simulink library "relay_modbus_lib"  (Simulink 8.1)
settings: Solver=ode45  StartTime=0.0  StopTime=10.0  RelTol=1e-3
undefined symbols (not defined in the file or in its folder): Ts
undefined symbols (not defined in the file): F4
libraries: simulink_extras x9, simulink x5, relay_PLL_lib x3, RMS_lib x3, powerlib_extras x2, relay_ANSI_functions_lib x2, relay_PQSPF_lib x1, relay_ANSI_F25_lib x1, relay_mgc_cmd_lib x1, relay_tripOutMng_lib x1
settings Model: Creator=RE25624  LastModifiedBy=hptb1

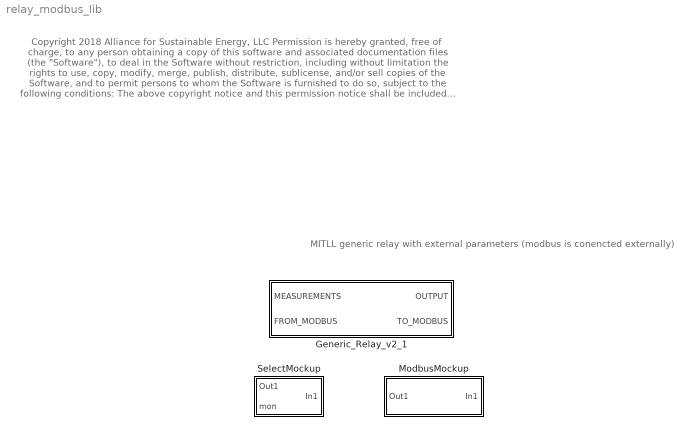
== system relay_modbus_lib ==
  note: MITLL generic relay with external parameters (modbus is conencted externally)
  note: Copyright 2018 Alliance for Sustainable Energy, LLC
      |
      | Permission is hereby granted, free of charge, to any person obtaining a copy of this software
      | and associated documentation files (the "Software"), to deal in the Software without restriction,
      | including without limitation the rights to use, copy, modify, merge, publish, distribute, sublicense,
      | and/or sell copies of the Software, and to permit persons to whom the Software is furnished to do so,
      | subject to the following conditions:
      |
      | The above copyright notice and this permission notice shall be included in all copies or substantial portions of the Software.
      |
      | THE SOFTWARE IS PROVIDED "AS IS", WITHOUT WARRANTY OF ANY KIND, EXPRESS OR IMPLIED, INCLUDING
      | BUT NOT LIMITED TO THE WARRANTIES OF MERCHANTABILITY, FITNESS FOR A PARTICULAR PURPOSE AND
      | NONINFRINGEMENT. IN NO EVENT SHALL THE AUTHORS, THE COPYRIGHT HOLDERS, THE UNITED STATES,
      | THE UNITED STATES DEPARTMENT OF ENERGY, OR ANY OF THEIR EMPLOYEES BE LIABLE FOR ANY CLAIM,
      | DAMAGES OR OTHER LIABILITY, WHETHER IN AN ACTION OF CONTRACT, TORT OR OTHERWISE, ARISING FROM,
      | OUT OF OR IN CONNECTION WITH THE SOFTWARE OR THE USE OR OTHER DEALINGS IN THE SOFTWARE.
  Generic_Relay_v2_1 : Subsystem  mask(Generic Relay){Ts=Ts, relay_settings=[F4(1,:)]}
      mask prompts: Ts "Sampling Time [Sec]"; relay_settings "Relay Settings"
      mask help:
      | This relay simulates functions: synchronizing or synchronism-check (25), phase instantaneous overcurrent (50P), AC inverse time overcurrent (51P), undervoltage relay (27), and overvoltage relay (59).
      |
      | FEATURES:
      | 1) Receives commands from the microgrid controller via MODBUS/TCP
      | 2) Two groups of interchangeable protection settings
      |     - To be used for grid-tied and islanded protection modes
      | 3) Locked-out only enabled for functions (50P), (51P)
      |     - (27) and (59) pickups will be model inputs for the next revision
      | 4) MODBUS commands expected in the following order:
      |    a) Functions reset (Holding Reg# 2000)
      |    b) Breaker state   (Holding Reg# 2001)
      |    c) Protection mode (Holding Reg# 2002)
      |       - bit = 0; parameter group#1 (default)
      |       - bit = 1; parameter group#2
      |
      | See help or integration packet for further information.
      mask Help:
      | Procedure to reclose a breaker:
      | 1) reset all functions (Holding Reg# 2000)
      | 2) set breaker state (Holding Reg# 2001) to generate a close signal
      | 	- Synch-check (25) will automatically activate
      | 	- bit = 0, trip functions are active
      | 	- bit = 1, trip functions are not active
      | 
      | 
      | 
      | Field format/order for relay settings:
      | 	- Assuming zero delay between group settings changes
      | 
      | 1.  Relay#
      | 2.  Nominal VRMSLL
      | 3.  Max. Slip Voltage [%]
      | 4.  Max. Slip Angle [degree]
      | 5.  Max. Slip Frequency [Hz]
      | 6.  27P and 59P Trip Delay [Sec]
      | 7.  CT Primary
      | 
      | Parameter Group #1
      | 8.  50P Instantaneous overcurrent (IOC) Trip Pickup
      | 9.  50P IOC Trip Delay [sec]
      | 10.  51P Time overcurrent (TOC) Trip Pickup
      | 11.  51P Curve Type
      | 12.  51P TOC Time Dial
      | 13.  27P Trip Pickup [pu]
      | 14.  59P Trip Pickup [pu]
      | 
      | Parameter Group #2
      | 15.  50P IOC Trip Pickup
      | 16.  50P IOC Trip Delay [sec]
      | 17.  51P TOC Trip Pickup
      | 18.  51P Curve Type
      | 19.  51P TOC Time Dial
      | 20.  27P Trip Pickup [pu]
      | 21.  59P Trip Pickup [pu]
      | 
      | Available TCC Characteristics:
      | 	- The degree of inverseness for each curve approximates SEL-751
      | 
      | 51P Curve
      | 1: moderate inverse
      | 2: inverse
      | 3: very inverse
      | 4: extremely inverse
      | 
      | References:
      | [1] IEEE Std. C37.112-1996
      | [2] SEL 751 Instruction manual
      | [3] MIT-LL 2nd Microgrid Controller Symposium - Integration Packet
  ModbusMockup : Subsystem
  SelectMockup : Subsystem  mask{sigID=1, sigN=6}
      mask prompts: sigID "Signal ID"; sigN "Signals count"
      mask Display: disp(['Select signal\n' num2str(sigID) '/' num2str(sigN)]);

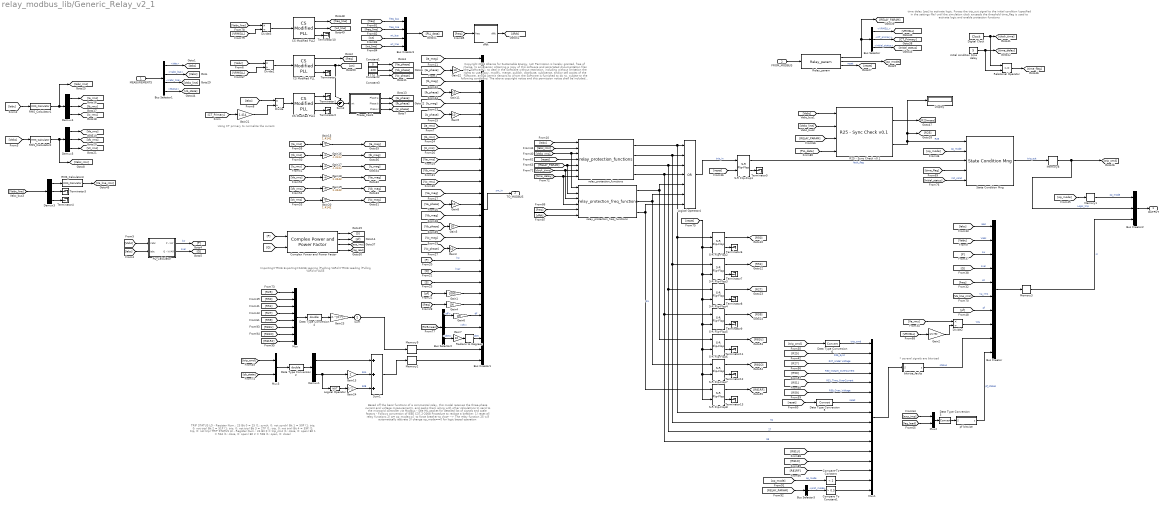
== system relay_modbus_lib/Generic_Relay_v2_1 ==
  note: Importing=TRUE
      | Exporting=FALSE
      |
      | Lagging (Pushing VARs)=TRUE
      | Leading (Pulling VARs)=FALSE
  note: * several signals are bitwised
  note: Using CT primary to normalize the current.
  note: TRIP STATUS LO - Register Num.: 23
      | Bit 0 = 25  (1: synch, 0: not synch)
      | Bit 1 = 50P (1: trip, 0: not trip)
      | Bit 2 = 51P (1: trip, 0: not trip)
      | Bit 3 = 27P (1: trip, 0: not trip)
      | Bit 4 = 59P (1: trip, 0: not trip)
      |
      | TRIP STATUS HI - Register Num.: 24
      | Bit 0 = trip_cmd  (1: close, 0: open)
      | Bit 1 = 52A (1: close, 0: open)
      | Bit 2 = 52B (1: open, 0: close)
  note: Based off the basic functions of a commercial relay, this model receives
      | the three-phase current and voltage measurements, and packs
      | them along with other calculations to send to the microgrid
      | controller via Modbus
      |
      | - See HIL packet for detailed list of signals and scale factors
      | - Follows convention of IEEE C37.2-2008
      |
      | Procedure to reclose a breaker:
      | 1) reset all relay functions
      | 2) set op_mode==1 to force breaker to close
      |    --> The relay function 25 will automatically activate
      | 3) change op_mode==0 for logic based operation
  note: time delay [sec] to activate logic. Forces the trip_out signal to the initial condition
      | (specified in the settings file) until the simulation clock exceeds the threshold
      |
      | time_flag is used to activate logic and enable protection functions
  note: Copyright 2018 Alliance for Sustainable Energy, LLC
      |
      | Permission is hereby granted, free of charge, to any person obtaining a copy of this software
      | and associated documentation files (the "Software"), to deal in the Software without restriction,
      | including without limitation the rights to use, copy, modify, merge, publish, distribute, sublicense,
      | and/or sell copies of the Software, and to permit persons to whom the Software is furnished to do so,
      | subject to the following conditions:
      |
      | The above copyright notice and this permission notice shall be included in all copies or substantial portions of the Software.
      |
      | THE SOFTWARE IS PROVIDED "AS IS", WITHOUT WARRANTY OF ANY KIND, EXPRESS OR IMPLIED, INCLUDING
      | BUT NOT LIMITED TO THE WARRANTIES OF MERCHANTABILITY, FITNESS FOR A PARTICULAR PURPOSE AND
      | NONINFRINGEMENT. IN NO EVENT SHALL THE AUTHORS, THE COPYRIGHT HOLDERS, THE UNITED STATES,
      | THE UNITED STATES DEPARTMENT OF ENERGY, OR ANY OF THEIR EMPLOYEES BE LIABLE FOR ANY CLAIM,
      | DAMAGES OR OTHER LIABILITY, WHETHER IN AN ACTION OF CONTRACT, TORT OR OTHERWISE, ARISING FROM,
      | OUT OF OR IN CONNECTION WITH THE SOFTWARE OR THE USE OR OTHER DEALINGS IN THE SOFTWARE.
  MEASUREMENTS : Inport
  FROM_MODBUS : Inport  Port=2
  Bus Creator : BusCreator  Inputs=10
  Bus Creator1 : BusCreator  Inputs=28
  Bus Creator2 : BusCreator  Inputs=3
  Bus Creator3 : BusCreator
  Bus Selector : BusSelector  OutputSignals=VRMSLL,CT_primary,Initial_status
  Bus Selector1 : BusSelector  OutputSignals=Iabc,Vabc_bus,Vabc_line,Status
  Bus Selector2 : BusSelector  OutputSignals=dF,dV,dWt
  Bus Selector3 : BusSelector  OutputSignals=prot_mode
  CS Modified PLL : relay_PLL_lib/CS Modified PLL  Flim=[55 66]  Par_Init=[0 60]  ParK=[ 180 3200 1 ]  Ts=Ts  AGC=off
  CS Modified PLL1 : relay_PLL_lib/CS Modified PLL  Flim=[55 66]  Par_Init=[0 60]  ParK=[ 180 3200 1 ]  Ts=Ts  AGC=off
  CS Modified PLL2 : relay_PLL_lib/CS Modified PLL  Flim=[55 66]  Par_Init=[0 60]  ParK=[ 180 3200 1 ]  Ts=Ts  AGC=off
  Compare To Constant : simulink/Logic and Bit Operations/Compare To Constant  relop=<  const=2  OutDataTypeStr=boolean
  Compare To Constant1 : simulink/Logic and Bit Operations/Compare To Constant  relop=>  const=0.5  OutDataTypeStr=boolean
  Complex Power and Power Factor : relay_PQSPF_lib/Complex Power and Power Factor
  Constant1 : Constant  Value=0
  Constant2 : Constant  Value=-120
  Constant3 : Constant  Value=120
  Data Type Conversion2 : DataTypeConversion  OutDataTypeStr=double
  Data Type Conversion3 : DataTypeConversion
  Data Type Conversion4 : DataTypeConversion  OutDataTypeStr=double
  Data Type Conversion5 : DataTypeConversion
  Data Type Conversion6 : DataTypeConversion
  Demux1 : Demux  Outputs=2
  Demux3 : Demux  Outputs=3
  Demux4 : Demux  Outputs=3
  Demux5 : Demux  Outputs=3
  Digital Clock : DigitalClock  SampleTime=Ts
  Display : Display
  Divide{,1..3} (4 alike) : Product  Inputs=*/
  Gain1 : Gain  Gain=1000
  Gain{3,5,7..9,11..12} (7 alike) : Gain  Gain=10
  Gain13 : Gain  Gain=2
  Gain{15..20} (6 alike) : Gain  Gain=1.4142
  Gain2 : Gain  Gain=1/1.732
  Gain21 : Gain  Gain=1.414
  Gain23 : Gain  Gain=2.^[0:7]
  Gain24 : Gain  Gain=2^2
  Gain4 : Gain  Gain=100
  Gain6 : Gain  Gain=100
  Logical Operator : Logic  Operator=NOT  AllPortsSameDT=off  OutDataTypeStr=boolean
  Logical Operator4 : Logic  Operator=OR  Inputs=7  AllPortsSameDT=off  OutDataTypeStr=boolean
  Memory{1..3,8..9} (5 alike) : Memory
  Mux : Mux  Inputs=8
  Mux1 : Mux  Inputs=16
  Mux2 : Mux  Inputs=2
  Mux3 : Mux  Inputs=2
  PQ_Calculator : Subsystem
  Phase_Calc1 : Subsystem
  R25 - Sync Check v0.1 : relay_ANSI_F25_lib/R25 - Sync Check v0.1  Ts=Ts
  RMS_Calculator1 : RMS_lib/RMS_Calculator  Ts=Ts
  RMS_Calculator2 : RMS_lib/RMS_Calculator  Ts=Ts
  RMS_Calculator3 : RMS_lib/RMS_Calculator  Ts=Ts
  Radians to Degrees : simulink_extras/Transformations/Radians to Degrees
  Relational Operator : RelationalOperator  OutDataTypeStr=boolean
  Relay_param : relay_mgc_cmd_lib/Relay_param  relay_settings=relay_settings
  S-R Flip-Flop{1..8} (8 alike) : simulink_extras/Flip Flops/S-R Flip-Flop  initial_condition=0
  State Condition Mng : relay_tripOutMng_lib/State Condition Mng
  Sum : Sum  Inputs=+
  Sum1 : Sum  Inputs=+++
  Sum2 : Sum  Inputs=-+|
  Terminator{,1..13} (14 alike) : Terminator
  bitwise_faults : Subsystem
  dfdt : Subsystem
  initial condition time delay : Constant  Value=5
  pf bitwise : Subsystem
  relay_protection_freq_functions : relay_ANSI_functions_lib/relay_protection_freq_functions  Ts=Ts
  relay_protection_functions : relay_ANSI_functions_lib/relay_protection_functions  Ts=Ts
  OUTPUT : Outport
  TO_MODBUS : Outport  Port=2
  wires:
  Gain23/1 -> Sum/1
  [R81RF] -> Mux/8
  [R81O] -> Mux/7
  [R81U] -> Mux/6
  Compare To Constant1/1 -> Mux1/16
  Bus Selector3/1 -> Compare To Constant1/1  "<prot_mode>"
  [RELAY_PARAM] -> Bus Selector3/1
  Compare To Constant/1 -> Mux1/15
  [op_mode] -> Compare To Constant/1  "op_mode"
  [R81RF] -> Mux1/14
  [R81O] -> Mux1/13
  [R81U] -> Mux1/12
  relay_protection_freq_functions/2 -> S-R Flip-Flop7/1, Logical Operator4/6
  relay_protection_freq_functions/1 -> Logical Operator4/5, S-R Flip-Flop6/1
  S-R Flip-Flop6/1 -> [R81U]
  S-R Flip-Flop7/1 -> [R81O]
  S-R Flip-Flop8/1 -> [R81RF]
  S-R Flip-Flop8/2 -> Terminator13/1
  S-R Flip-Flop7/2 -> Terminator12/1
  S-R Flip-Flop6/2 -> Terminator11/1
  [reset] -> S-R Flip-Flop2/2, S-R Flip-Flop3/2, S-R Flip-Flop4/2, S-R Flip-Flop5/2, S-R Flip-Flop6/2, S-R Flip-Flop7/2, S-R Flip-Flop8/2
  relay_protection_freq_functions/3 -> Logical Operator4/7, S-R Flip-Flop8/1  "51"
  [dfdt] -> relay_protection_freq_functions/6
  [freq] -> relay_protection_freq_functions/5
  dfdt/1(dfdt) -> [dfdt]
  [freq] -> dfdt/1(freq)
  [wt_line] -> Bus Creator3/4  "wt_line"
  [wt] -> Bus Creator3/3  "wt_bus"
  [freq_line] -> Bus Creator3/2  "freq_line"
  [freq] -> Bus Creator3/1  "freq_bus"
  Bus Creator3/1 -> [PLL_data]
  [PLL_data] -> R25 - Sync Check v0.1/4
  CS Modified PLL2/3 -> Terminator10/1
  CS Modified PLL2/2 -> [wt_line]
  CS Modified PLL2/1 -> [freq_line]
  Divide3/1 -> CS Modified PLL2/1
  [VRMSLL] -> Divide3/2
  [Vabc_line] -> Divide3/1
  Radians to Degrees/1 -> Bus Creator1/26  "dWt"
  Gain7/1 -> Radians to Degrees/1
  Gain6/1 -> Bus Creator1/24  "dF"
  Bus Selector2/3 -> Gain7/1  "<dWt>"
  Bus Selector2/1 -> Gain6/1  "<dF>"
  Bus Selector2/2 -> Bus Creator1/25  "<dV>"
  [R25meas] -> Bus Selector2/1
  R25 - Sync Check v0.1/1 -> [R25meas]
  relay_protection_functions/1 -> Logical Operator4/1, S-R Flip-Flop2/1, Mux1/8
  [S] -> Bus Creator1/21
  [Q] -> Bus Creator1/20  "kvar"
  [P] -> Bus Creator1/19  "kw"
  Sum2/1 -> Phase_Calc1/1(wt)
  S-R Flip-Flop2/1 -> [R50]
  S-R Flip-Flop3/1 -> [R51]
  S-R Flip-Flop4/1 -> [R27]
  S-R Flip-Flop5/1 -> [R59]
  S-R Flip-Flop5/2 -> Terminator9/1
  S-R Flip-Flop4/2 -> Terminator8/1
  S-R Flip-Flop3/2 -> Terminator7/1
  S-R Flip-Flop2/2 -> Terminator6/1
  RMS_Calculator3/1 -> [Va_line_rms]
  [Vabc_line] -> Demux3/1
  Relational Operator/1 -> [time_flag]
  Demux3/3 -> Terminator4/1
  Demux3/2 -> Terminator3/1
  Demux3/1 -> RMS_Calculator3/1
  Gain2/1 -> Divide2/2
  Logical Operator/1 -> Gain24/1
  [Initial_status] -> State Condition Mng/5  "init_cond"
  Bus Selector/3 -> [Initial_status]  "<Initial_status>"
  [time_delay] -> relay_protection_freq_functions/4, relay_protection_functions/7
  [clock_time] -> relay_protection_freq_functions/3, relay_protection_functions/6
  Relay_param/3 -> [reset]  "reset"
  initial condition time delay/1 -> [time_delay], Relational Operator/2
  [time_flag] -> State Condition Mng/4
  Digital Clock/1 -> [clock_time], Relational Operator/1
  Gain21/1 -> Divide/2
  Relay_param/2 -> [op_mode]
  [Va_rms] -> Divide2/1
  [VRMSLL] -> Gain2/1
  [VRMSLL] -> Divide1/2
  Divide1/1 -> CS Modified PLL/1
  [Vabc] -> Divide1/1
  Bus Selector/1 -> [VRMSLL]  "<VRMSLL>"
  [RELAY_PARAM] -> R25 - Sync Check v0.1/3
  [RELAY_PARAM] -> relay_protection_freq_functions/2, relay_protection_functions/5
  [Iabc] -> relay_protection_functions/1
  [Vabc_rms] -> relay_protection_freq_functions/1, relay_protection_functions/3
  [Iabc_rms] -> relay_protection_functions/2
  [reset] -> relay_protection_functions/4
  Relay_param/1 -> Bus Selector/1, [RELAY_PARAM]
  Bus Selector/2 -> [CT_Primary]  "<CT_primary>"
  Data Type Conversion3/1 -> pf bitwise/1(S)
  Memory3/1 -> Bus Creator2/3  "m"
  [lag_lead] -> Mux2/2
  [exp_imp] -> Mux2/1
  pf bitwise/1(s) -> Bus Creator/10  "pf_states"
  Mux2/1 -> Data Type Conversion3/1
  Complex Power and Power Factor/4 -> [lag_lead]
  Complex Power and Power Factor/3 -> [exp_imp]
  Complex Power and Power Factor/2 -> [pf]
  Complex Power and Power Factor/1 -> [S]
  [Q] -> Complex Power and Power Factor/2
  [P] -> Complex Power and Power Factor/1
  Bus Creator2/1 -> OUTPUT/1
  Memory1/1 -> Bus Creator2/1  "op_mode"
  Bus Creator/1 -> Memory3/1
  MEASUREMENTS/1 -> Bus Selector1/1
  Bus Selector1/3 -> [Vabc_line]  "<Vabc_line>"
  Bus Selector1/2 -> [Vabc]  "<Vabc_bus>"
  Bus Selector1/1 -> [Iabc]  "<Iabc>"
  [Vabc_line] -> R25 - Sync Check v0.1/2
  Data Type Conversion6/1 -> Mux1/1  "trip_cmd"
  Data Type Conversion5/1 -> Mux1/7  "reset"
  [R59] -> Mux1/6  "R59_Over_Voltage"
  [R51] -> Mux1/5  "R51_Time_OverCurrent"
  [R50] -> Mux1/4  "R50_Instant_OverCurrent"
  [R27] -> Mux1/3  "R27_Under Voltage"
  [R25] -> Mux1/2  "R25_Sync"
  [trip_cmd] -> Data Type Conversion6/1
  [reset] -> Data Type Conversion5/1
  bitwise_faults/1(s) -> Bus Creator/9  "status"
  Mux1/1 -> bitwise_faults/1(S)
  relay_protection_functions/4 -> Logical Operator4/4, S-R Flip-Flop5/1, Mux1/11  "59"
  relay_protection_functions/3 -> Logical Operator4/3, S-R Flip-Flop4/1, Mux1/10  "27"
  Divide2/1 -> Bus Creator/8  "Vpu"
  Gain15/1 -> [Ia_mag]
  Gain16/1 -> [Ib_mag]
  Gain17/1 -> [Ic_mag]
  Gain18/1 -> [Va_mag]
  Gain19/1 -> [Vb_mag]
  Gain20/1 -> [Vc_mag]
  [Vc_rms] -> Gain20/1
  [Vb_rms] -> Gain19/1
  [Va_rms] -> Gain18/1
  [Ic_rms] -> Gain17/1
  [Ib_rms] -> Gain16/1
  [Ia_rms] -> Gain15/1
  [Vabc] -> R25 - Sync Check v0.1/1
  Gain4/1 -> Bus Creator1/23
  Gain1/1 -> Bus Creator1/22
  Gain3/1 -> Bus Creator1/18
  [Vc_mag] -> Bus Creator1/17
  Gain5/1 -> Bus Creator1/16
  [Vb_mag] -> Bus Creator1/15
  Gain8/1 -> Bus Creator1/14
  [Va_mag] -> Bus Creator1/13
  [Vc_rms] -> Bus Creator1/12
  [Vb_rms] -> Bus Creator1/11
  [Va_rms] -> Bus Creator1/10
  [Ic_rms] -> Bus Creator1/9
  [Ib_rms] -> Bus Creator1/8
  [Ia_rms] -> Bus Creator1/7
  Gain9/1 -> Bus Creator1/6
  [Ic_mag] -> Bus Creator1/5
  Gain11/1 -> Bus Creator1/4
  [Ib_mag] -> Bus Creator1/3
  Gain12/1 -> Bus Creator1/2
  [Ia_mag] -> Bus Creator1/1
  [pf] -> Bus Creator/7  "pf"
  [Va_line_rms] -> Bus Creator/6  "Va_rms"
  [freq] -> Bus Creator/5  "Hz"
  CS Modified PLL/3 -> Terminator/1
  CS Modified PLL1/3 -> Terminator2/1
  CS Modified PLL1/1 -> Terminator1/1
  CS Modified PLL/2 -> Sum2/1, [wt]
  CS Modified PLL/1 -> [freq]
  CS Modified PLL1/2 -> Sum2/2
  S-R Flip-Flop1/1 -> State Condition Mng/3  "fault_flag"
  [op_mode] -> State Condition Mng/2  "op_mode"
  R25 - Sync Check v0.1/2 -> State Condition Mng/1, [R25], Display/1  "R25"
  Memory8/1 -> Bus Creator2/2, [trip_cmd]  "Logic_trip"
  [op_mode] -> Memory1/1
  Memory2/1 -> Bus Creator1/28
  Memory9/1 -> Bus Creator1/27
  Data Type Conversion4/1 -> Gain23/1
  Mux/1 -> Data Type Conversion4/1
  relay_protection_functions/2 -> Logical Operator4/2, S-R Flip-Flop3/1, Mux1/9  "51"
  Sum/1 -> Memory9/1
  Sum1/1 -> Memory2/1
  [Ia_phase] -> Gain12/1
  [Ib_phase] -> Gain11/1
  [Ic_phase] -> Gain9/1
  [Va_phase] -> Gain8/1
  [Vb_phase] -> Gain5/1
  [Vc_phase] -> Gain3/1
  [CT_Primary] -> Gain21/1
  Divide/1 -> CS Modified PLL1/1
  Phase_Calc1/3(Phase c) -> [Ic_phase]
  Phase_Calc1/2(Phase b) -> [Ib_phase]
  Phase_Calc1/1(Phase a) -> [Ia_phase]
  [Iabc] -> Divide/1
  Constant3/1 -> [Vc_phase]
  Constant2/1 -> [Vb_phase]
  Constant1/1 -> [Va_phase]
  [Q] -> Bus Creator/4  "kvar"
  [P] -> Bus Creator/3  "kw"
  [pf] -> Gain1/1
  [freq] -> Gain4/1
  Bus Creator1/1 -> TO_MODBUS/1  "sm_in"
  FROM_MODBUS/1 -> Relay_param/1
  [Vabc] -> Bus Creator/2  "Vabc"
  [Iabc] -> Bus Creator/1  "Iabc"
  [Vabc] -> PQ_Calculator/1(Vabc)
  [Iabc] -> PQ_Calculator/2(Iabc)
  PQ_Calculator/1(P - kW) -> [P]  "kw"
  PQ_Calculator/2(Q - kVAR) -> [Q]  "kvar"
  [Iabc] -> RMS_Calculator1/1
  [Vabc] -> RMS_Calculator2/1
  RMS_Calculator1/1 -> Demux4/1, [Iabc_rms]
  RMS_Calculator2/1 -> Demux5/1, [Vabc_rms]
  Demux4/3 -> [Ic_rms]
  Demux4/2 -> [Ib_rms]
  Demux4/1 -> [Ia_rms]
  Demux5/1 -> [Va_rms]
  Demux5/2 -> [Vb_rms]
  Demux5/3 -> [Vc_rms]
  State Condition Mng/1 -> Memory8/1  "trip_out"
  Bus Selector1/4 -> [cb_state]  "<Status>"
  [R25] -> Mux/1
  [R50] -> Mux/2
  [R51] -> Mux/3
  [R27] -> Mux/4
  [R59] -> Mux/5
  Mux3/1 -> Data Type Conversion2/1
  Gain13/1 -> Sum1/2  "52A"
  Demux1/1 -> Sum1/1
  Data Type Conversion2/1 -> Demux1/1
  [trip_cmd] -> Mux3/1
  [cb_state] -> Mux3/2
  Gain24/1 -> Sum1/3  "52B"
  Demux1/2 -> Logical Operator/1, Gain13/1
  S-R Flip-Flop1/2 -> Terminator5/1
  [reset] -> S-R Flip-Flop1/2
  Logical Operator4/1 -> S-R Flip-Flop1/1  "trip_in"

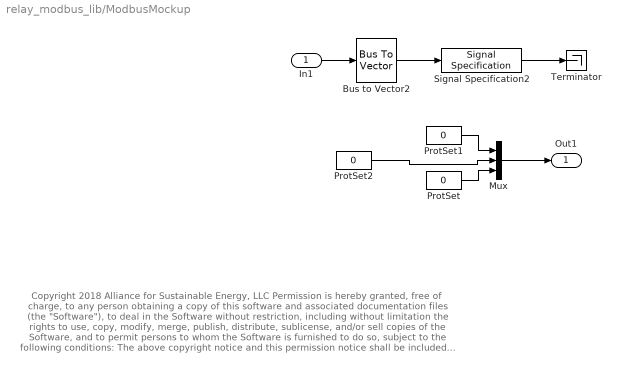
== system relay_modbus_lib/ModbusMockup ==
  note: Copyright 2018 Alliance for Sustainable Energy, LLC
      |
      | Permission is hereby granted, free of charge, to any person obtaining a copy of this software
      | and associated documentation files (the "Software"), to deal in the Software without restriction,
      | including without limitation the rights to use, copy, modify, merge, publish, distribute, sublicense,
      | and/or sell copies of the Software, and to permit persons to whom the Software is furnished to do so,
      | subject to the following conditions:
      |
      | The above copyright notice and this permission notice shall be included in all copies or substantial portions of the Software.
      |
      | THE SOFTWARE IS PROVIDED "AS IS", WITHOUT WARRANTY OF ANY KIND, EXPRESS OR IMPLIED, INCLUDING
      | BUT NOT LIMITED TO THE WARRANTIES OF MERCHANTABILITY, FITNESS FOR A PARTICULAR PURPOSE AND
      | NONINFRINGEMENT. IN NO EVENT SHALL THE AUTHORS, THE COPYRIGHT HOLDERS, THE UNITED STATES,
      | THE UNITED STATES DEPARTMENT OF ENERGY, OR ANY OF THEIR EMPLOYEES BE LIABLE FOR ANY CLAIM,
      | DAMAGES OR OTHER LIABILITY, WHETHER IN AN ACTION OF CONTRACT, TORT OR OTHERWISE, ARISING FROM,
      | OUT OF OR IN CONNECTION WITH THE SOFTWARE OR THE USE OR OTHER DEALINGS IN THE SOFTWARE.
  In1 : Inport
  Bus to Vector2 : BusToVector
  Mux : Mux  Inputs=3
  ProtSet : Constant  Value=0
  ProtSet1 : Constant  Value=0
  ProtSet2 : Constant  Value=0
  Signal Specification2 : SignalSpecification  OutDataTypeStr=double  Dimensions=25
  Terminator : Terminator
  Out1 : Outport
  wires:
  In1/1 -> Bus to Vector2/1
  Bus to Vector2/1 -> Signal Specification2/1
  ProtSet2/1 -> Mux/2
  ProtSet1/1 -> Mux/1
  ProtSet/1 -> Mux/3
  Mux/1 -> Out1/1
  Signal Specification2/1 -> Terminator/1

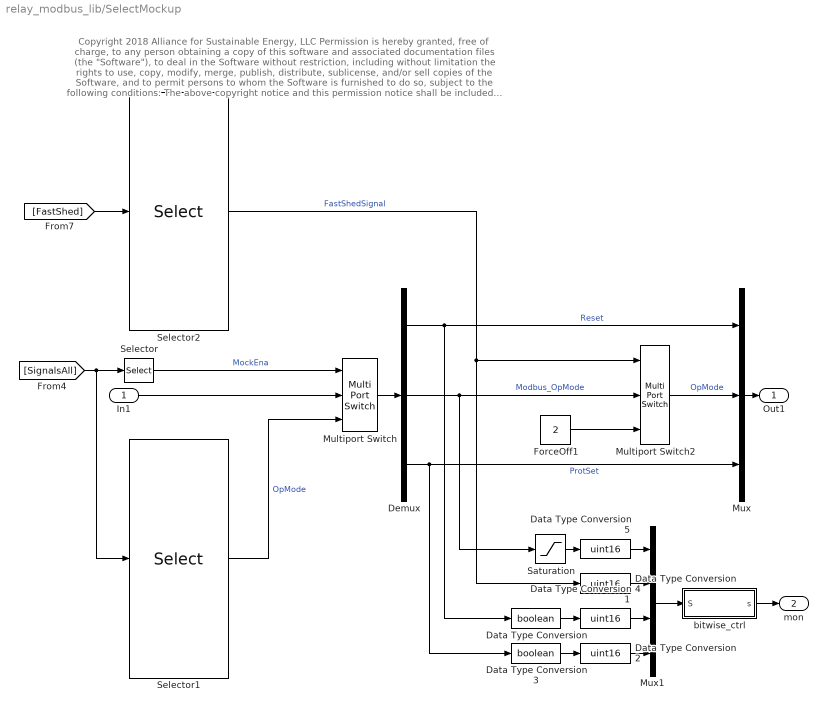
== system relay_modbus_lib/SelectMockup ==
  note: Copyright 2018 Alliance for Sustainable Energy, LLC
      |
      | Permission is hereby granted, free of charge, to any person obtaining a copy of this software
      | and associated documentation files (the "Software"), to deal in the Software without restriction,
      | including without limitation the rights to use, copy, modify, merge, publish, distribute, sublicense,
      | and/or sell copies of the Software, and to permit persons to whom the Software is furnished to do so,
      | subject to the following conditions:
      |
      | The above copyright notice and this permission notice shall be included in all copies or substantial portions of the Software.
      |
      | THE SOFTWARE IS PROVIDED "AS IS", WITHOUT WARRANTY OF ANY KIND, EXPRESS OR IMPLIED, INCLUDING
      | BUT NOT LIMITED TO THE WARRANTIES OF MERCHANTABILITY, FITNESS FOR A PARTICULAR PURPOSE AND
      | NONINFRINGEMENT. IN NO EVENT SHALL THE AUTHORS, THE COPYRIGHT HOLDERS, THE UNITED STATES,
      | THE UNITED STATES DEPARTMENT OF ENERGY, OR ANY OF THEIR EMPLOYEES BE LIABLE FOR ANY CLAIM,
      | DAMAGES OR OTHER LIABILITY, WHETHER IN AN ACTION OF CONTRACT, TORT OR OTHERWISE, ARISING FROM,
      | OUT OF OR IN CONNECTION WITH THE SOFTWARE OR THE USE OR OTHER DEALINGS IN THE SOFTWARE.
  In1 : Inport
  Data Type Conversion : DataTypeConversion  OutDataTypeStr=boolean
  Data Type Conversion{1..2,4..5} (4 alike) : DataTypeConversion  OutDataTypeStr=uint16
  Data Type Conversion3 : DataTypeConversion  OutDataTypeStr=boolean
  Demux : Demux  Outputs=3
  ForceOff1 : Constant  Value=2
  Multiport Switch : MultiPortSwitch  DataPortOrder=Zero-based contiguous  Inputs=2
  Multiport Switch2 : MultiPortSwitch  DataPortOrder=Zero-based contiguous  Inputs=2
  Mux : Mux  Inputs=3
  Mux1 : Mux
  Saturation : Saturate  UpperLimit=3  LowerLimit=0
  Selector : Selector  InputPortWidth=sigN+3  IndexOptions=Index vector (dialog)  Indices=[1]  OutputSizes=1
  Selector1 : Selector  InputPortWidth=sigN+3  IndexOptions=Index vector (dialog)  Indices="[2  sigID+3 3]"  OutputSizes=1
  Selector2 : Selector  InputPortWidth=sigN  IndexOptions=Index vector (dialog)  Indices=[sigID]  OutputSizes=1
  bitwise_ctrl : Subsystem
  Out1 : Outport
  mon : Outport  Port=2
  wires:
  Selector2/1 -> Multiport Switch2/1, Data Type Conversion4/1  "FastShedSignal"
  Demux/2 -> Multiport Switch2/2, Saturation/1  "Modbus_OpMode"
  Demux/3 -> Mux/3, Data Type Conversion3/1  "ProtSet"
  Demux/1 -> Mux/1, Data Type Conversion/1  "Reset"
  Mux1/1 -> bitwise_ctrl/1(S)
  bitwise_ctrl/1(s) -> mon/1
  Saturation/1 -> Data Type Conversion5/1
  Data Type Conversion/1 -> Data Type Conversion1/1
  Data Type Conversion1/1 -> Mux1/3
  Data Type Conversion2/1 -> Mux1/4
  Data Type Conversion3/1 -> Data Type Conversion2/1
  Data Type Conversion4/1 -> Mux1/2
  Data Type Conversion5/1 -> Mux1/1
  ForceOff1/1 -> Multiport Switch2/3
  Multiport Switch2/1 -> Mux/2  "OpMode"
  Mux/1 -> Out1/1
  [FastShed] -> Selector2/1
  Multiport Switch/1 -> Demux/1
  In1/1 -> Multiport Switch/2
  [SignalsAll] -> Selector1/1, Selector/1
  Selector/1 -> Multiport Switch/1  "MockEna"
  Selector1/1 -> Multiport Switch/3  "OpMode"

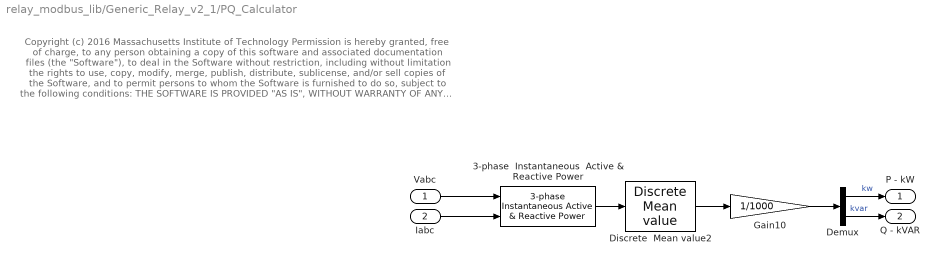
== system relay_modbus_lib/Generic_Relay_v2_1/PQ_Calculator ==
  note: Copyright (c) 2016 Massachusetts Institute of Technology
      | Permission is hereby granted, free of charge, to any person obtaining a copy of this software and associated documentation files (the "Software"), to deal
      | in the Software without restriction, including without limitation the rights to use, copy, modify, merge, publish, distribute, sublicense, and/or sell copies of the
      | Software, and to permit persons to whom the Software is furnished to do so, subject to the following conditions:
      |
      | THE SOFTWARE IS PROVIDED "AS IS", WITHOUT WARRANTY OF ANY KIND, EXPRESS OR IMPLIED, INCLUDING BUT NOT LIMITED TO THE
      | WARRANTIES OF MERCHANTABILITY, FITNESS FOR A PARTICULAR PURPOSE AND NONINFRINGEMENT. IN NO EVENT SHALL THE AUTHORS
      | OR COPYRIGHT HOLDERS BE LIABLE FOR ANY CLAIM, DAMAGES OR OTHER LIABILITY, WHETHER IN AN ACTION OF CONTRACT, TORT OR
      | OTHERWISE, ARISING FROM, OUT OF OR IN CONNECTION WITH THE SOFTWARE OR THE USE OR OTHER DEALINGS IN THE SOFTWARE
  Vabc : Inport
  Iabc : Inport  Port=2
  3-phase  Instantaneous  Active & Reactive Power : powerlib_extras/Measurements/3-phase  Instantaneous  Active & Reactive Power
  Demux : Demux  Outputs=2
  Discrete  Mean value2 : powerlib_extras/Discrete Measurements/Discrete  Mean value  Freq=60  Vinit=0  Ts=Ts
  Gain10 : Gain  Gain=1/1000
  P - kW : Outport
  Q - kVAR : Outport  Port=2
  wires:
  Gain10/1 -> Demux/1
  3-phase  Instantaneous  Active & Reactive Power/1 -> Discrete  Mean value2/1
  Discrete  Mean value2/1 -> Gain10/1
  Vabc/1 -> 3-phase  Instantaneous  Active & Reactive Power/1
  Iabc/1 -> 3-phase  Instantaneous  Active & Reactive Power/2
  Demux/1 -> P - kW/1  "kw"
  Demux/2 -> Q - kVAR/1  "kvar"

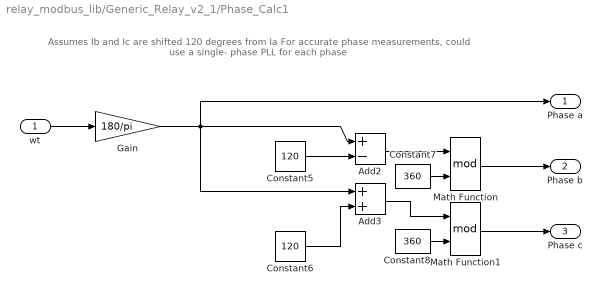
== system relay_modbus_lib/Generic_Relay_v2_1/Phase_Calc1 ==
  note: Assumes Ib and Ic are shifted 120 degrees from Ia
      | For accurate phase measurements, could use a single-
      | phase PLL for each phase
  wt : Inport
  Add2 : Sum  Inputs=+-
  Add3 : Sum
  Constant5 : Constant  Value=120
  Constant6 : Constant  Value=120
  Constant7 : Constant  Value=360
  Constant8 : Constant  Value=360
  Gain : Gain  Gain=180/pi
  Math Function : Math  Operator=mod  SaturateOnIntegerOverflow=on
  Math Function1 : Math  Operator=mod  SaturateOnIntegerOverflow=on
  Phase a : Outport
  Phase b : Outport  Port=2
  Phase c : Outport  Port=3
  wires:
  Constant5/1 -> Add2/2
  Constant6/1 -> Add3/2
  wt/1 -> Gain/1
  Constant7/1 -> Math Function/2
  Add2/1 -> Math Function/1
  Add3/1 -> Math Function1/1
  Constant8/1 -> Math Function1/2
  Math Function/1 -> Phase b/1
  Math Function1/1 -> Phase c/1
  Gain/1 -> Add3/1, Phase a/1, Add2/1

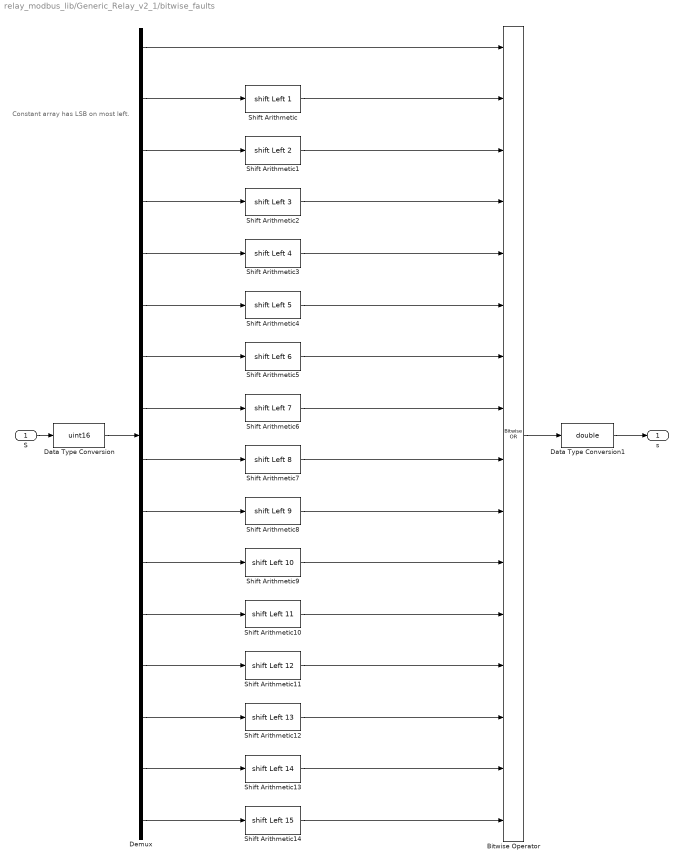
== system relay_modbus_lib/Generic_Relay_v2_1/bitwise_faults ==
  note: Constant array has LSB on most left.
  S : Inport
  Bitwise Operator : simulink/Logic and Bit Operations/Bitwise Operator  logicop=OR  UseBitMask=off  NumInputPorts=16  BitMask=bin2dec('11011001')  BitMaskRealWorld=Stored Integer
  Data Type Conversion : DataTypeConversion  OutDataTypeStr=uint16
  Data Type Conversion1 : DataTypeConversion  OutDataTypeStr=double
  Demux : Demux  Outputs=16
  Shift Arithmetic : ArithShift  BitShiftNumber=1  BitShiftDirection=Left
  Shift Arithmetic1 : ArithShift  BitShiftNumber=2  BitShiftDirection=Left
  Shift Arithmetic10 : ArithShift  BitShiftNumber=11  BitShiftDirection=Left
  Shift Arithmetic11 : ArithShift  BitShiftNumber=12  BitShiftDirection=Left
  Shift Arithmetic12 : ArithShift  BitShiftNumber=13  BitShiftDirection=Left
  Shift Arithmetic13 : ArithShift  BitShiftNumber=14  BitShiftDirection=Left
  Shift Arithmetic14 : ArithShift  BitShiftNumber=15  BitShiftDirection=Left
  Shift Arithmetic2 : ArithShift  BitShiftNumber=3  BitShiftDirection=Left
  Shift Arithmetic3 : ArithShift  BitShiftNumber=4  BitShiftDirection=Left
  Shift Arithmetic4 : ArithShift  BitShiftNumber=5  BitShiftDirection=Left
  Shift Arithmetic5 : ArithShift  BitShiftNumber=6  BitShiftDirection=Left
  Shift Arithmetic6 : ArithShift  BitShiftNumber=7  BitShiftDirection=Left
  Shift Arithmetic7 : ArithShift  BitShiftNumber=8  BitShiftDirection=Left
  Shift Arithmetic8 : ArithShift  BitShiftNumber=9  BitShiftDirection=Left
  Shift Arithmetic9 : ArithShift  BitShiftNumber=10  BitShiftDirection=Left
  s : Outport
  wires:
  Shift Arithmetic14/1 -> Bitwise Operator/16
  Shift Arithmetic13/1 -> Bitwise Operator/15
  Shift Arithmetic12/1 -> Bitwise Operator/14
  Shift Arithmetic11/1 -> Bitwise Operator/13
  Shift Arithmetic10/1 -> Bitwise Operator/12
  Demux/16 -> Shift Arithmetic14/1
  Demux/15 -> Shift Arithmetic13/1
  Demux/14 -> Shift Arithmetic12/1
  Demux/13 -> Shift Arithmetic11/1
  Demux/12 -> Shift Arithmetic10/1
  Demux/11 -> Shift Arithmetic9/1
  Demux/10 -> Shift Arithmetic8/1
  Demux/9 -> Shift Arithmetic7/1
  Demux/8 -> Shift Arithmetic6/1
  Shift Arithmetic7/1 -> Bitwise Operator/9
  Shift Arithmetic8/1 -> Bitwise Operator/10
  Shift Arithmetic6/1 -> Bitwise Operator/8
  Shift Arithmetic9/1 -> Bitwise Operator/11
  Shift Arithmetic5/1 -> Bitwise Operator/7
  Shift Arithmetic4/1 -> Bitwise Operator/6
  Shift Arithmetic3/1 -> Bitwise Operator/5
  Shift Arithmetic2/1 -> Bitwise Operator/4
  Shift Arithmetic1/1 -> Bitwise Operator/3
  Shift Arithmetic/1 -> Bitwise Operator/2
  Demux/7 -> Shift Arithmetic5/1
  Demux/6 -> Shift Arithmetic4/1
  Demux/5 -> Shift Arithmetic3/1
  Demux/4 -> Shift Arithmetic2/1
  Demux/3 -> Shift Arithmetic1/1
  Demux/2 -> Shift Arithmetic/1
  Demux/1 -> Bitwise Operator/1
  Data Type Conversion1/1 -> s/1
  Bitwise Operator/1 -> Data Type Conversion1/1
  S/1 -> Data Type Conversion/1
  Data Type Conversion/1 -> Demux/1

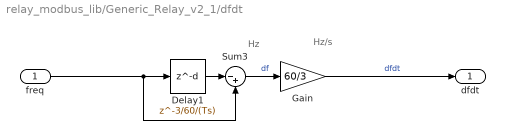
== system relay_modbus_lib/Generic_Relay_v2_1/dfdt ==
  note: Hz
  note: Hz/s
  freq : Inport
  Delay1 : Delay  DelayLength=3/60/(Ts)  UseCircularBuffer=on
  Gain : Gain  Gain=60/3
  Sum3 : Sum  Inputs=|-+
  dfdt : Outport
  wires:
  Gain/1 -> dfdt/1  "dfdt"
  Delay1/1 -> Sum3/1
  Sum3/1 -> Gain/1  "df"
  freq/1 -> Delay1/1, Sum3/2

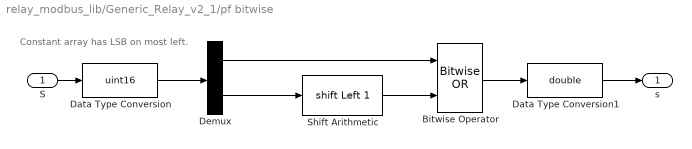
== system relay_modbus_lib/Generic_Relay_v2_1/pf bitwise ==
  note: Constant array has LSB on most left.
  S : Inport
  Bitwise Operator : simulink/Logic and Bit Operations/Bitwise Operator  logicop=OR  UseBitMask=off  NumInputPorts=2  BitMask=bin2dec('11011001')  BitMaskRealWorld=Stored Integer
  Data Type Conversion : DataTypeConversion  OutDataTypeStr=uint16
  Data Type Conversion1 : DataTypeConversion  OutDataTypeStr=double
  Demux : Demux  Outputs=2
  Shift Arithmetic : ArithShift  BitShiftNumber=1  BitShiftDirection=Left
  s : Outport
  wires:
  Data Type Conversion/1 -> Demux/1
  S/1 -> Data Type Conversion/1
  Bitwise Operator/1 -> Data Type Conversion1/1
  Data Type Conversion1/1 -> s/1
  Demux/1 -> Bitwise Operator/1
  Demux/2 -> Shift Arithmetic/1
  Shift Arithmetic/1 -> Bitwise Operator/2

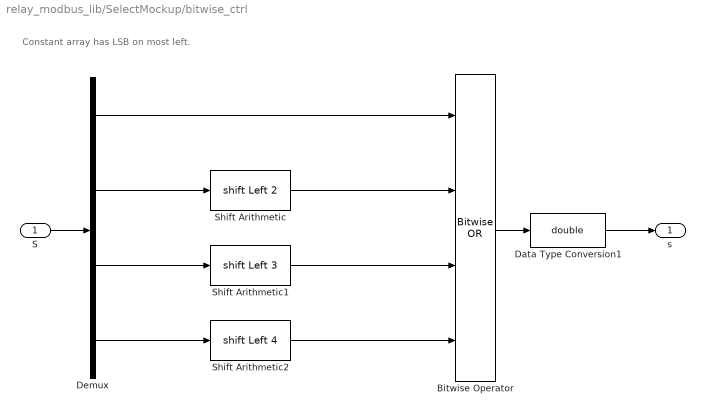
== system relay_modbus_lib/SelectMockup/bitwise_ctrl ==
  note: Constant array has LSB on most left.
  S : Inport
  Bitwise Operator : simulink/Logic and Bit Operations/Bitwise Operator  logicop=OR  UseBitMask=off  NumInputPorts=4  BitMask=bin2dec('11011001')  BitMaskRealWorld=Stored Integer
  Data Type Conversion1 : DataTypeConversion  OutDataTypeStr=double
  Demux : Demux
  Shift Arithmetic : ArithShift  BitShiftNumber=2  BitShiftDirection=Left
  Shift Arithmetic1 : ArithShift  BitShiftNumber=3  BitShiftDirection=Left
  Shift Arithmetic2 : ArithShift  BitShiftNumber=4  BitShiftDirection=Left
  s : Outport
  wires:
  Shift Arithmetic2/1 -> Bitwise Operator/4
  Shift Arithmetic1/1 -> Bitwise Operator/3
  Shift Arithmetic/1 -> Bitwise Operator/2
  Demux/4 -> Shift Arithmetic2/1
  Demux/3 -> Shift Arithmetic1/1
  Demux/2 -> Shift Arithmetic/1
  Demux/1 -> Bitwise Operator/1
  Data Type Conversion1/1 -> s/1
  Bitwise Operator/1 -> Data Type Conversion1/1
  S/1 -> Demux/1
